simulink model "elec_sys_isolated"  (R2013b)
settings: Solver=ode45  StartTime=0.0  StopTime=10.0  RelTol=1e-3
values from neighbouring files (symbols this model uses):
  avload =     [Benchmark_data1.mat]
libraries: PowerFlowLib x28, simulink x5
settings Model: Creator=srikanthan  LastModifiedBy=srikanthan

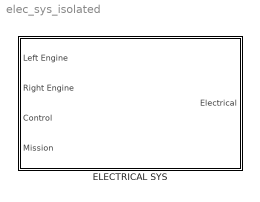
== system elec_sys_isolated ==
  "ELECTRICAL SYS " : Subsystem

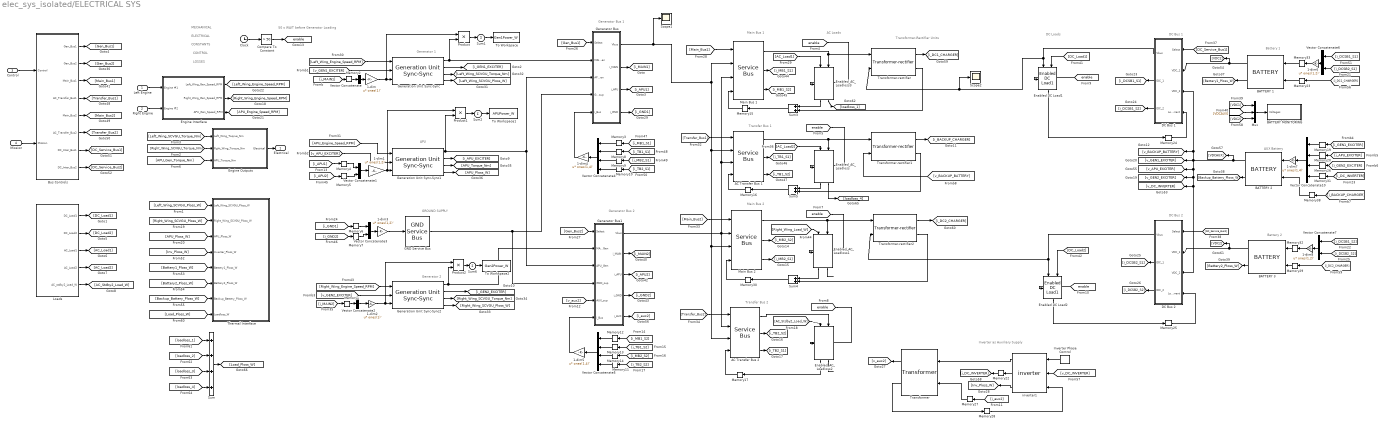
== system elec_sys_isolated/ELECTRICAL SYS  ==
  note: CONSTANTS
  note: CONTROL
  note: LOSSES
  note: MECHANICAL
  note: ELECTRICAL
  note: Generator Bus 1
  note: Generator 1
  note: APU
  note: GROUND SUPPLY
  note: Generator 2
  note: Main Bus 1
  note: Transfer Bus 1
  note: Main Bus 2
  note: Transfer Bus 2
  note: AC Loads
  note: Transformer-Rectifier Units
  note: DC Loads
  note: DC Bus 1
  note: DC Bus 2
  note: Battery 1
  note: AUX Battery
  note: Battery 2
  note: Inverter as Auxiliary Supply
  note: 50 s WAIT before Generator Loading
  note: Generator Bus 2
  Left Engine : Inport
  Right Engine : Inport  Port=2
  Control : Inport  Port=3
  Mission : Inport  Port=4
  " inverter1" : PowerFlowLib/Energy & Power Systems/Electrical/Inverters/ inverter  Trise=4e-6  Tfall=4e-6  fsw=2e3  Vcesat=1.2  Nofsw=6
  1-dim : Gain  Gain=ones(1)'  Multiplication=Matrix(u*K)
  1-dim{1,3,6,8} (4 alike) : Gain  Gain=ones(1,2)'  Multiplication=Matrix(u*K)
  1-dim2 : Gain  Gain=ones(1)'  Multiplication=Matrix(u*K)
  1-dim4 : Gain  Gain=ones(1,4)'  Multiplication=Matrix(u*K)
  1-dim5 : Gain  Gain=ones(1,4)'  Multiplication=Matrix(u*K)
  1-dim7 : Gain  Gain=ones(1,4)'  Multiplication=Matrix(u*K)
  AC Transfer Bus 1 : PowerFlowLib/Energy & Power Systems/Electrical/Systems/Service Bus
  AC Transfer Bus 2 : PowerFlowLib/Energy & Power Systems/Electrical/Systems/Service Bus
  BATTERY 1 : PowerFlowLib/Energy & Power Systems/Electrical/Battery/BATTERY  NO_CELLS=8  NO_MODULES=100  INITIAL_SOC=1
  BATTERY 2 : PowerFlowLib/Energy & Power Systems/Electrical/Battery/BATTERY  NO_CELLS=8  NO_MODULES=100  INITIAL_SOC=1
  BATTERY 3 : PowerFlowLib/Energy & Power Systems/Electrical/Battery/BATTERY  NO_CELLS=8  NO_MODULES=100  INITIAL_SOC=1
  BATTERY MONITORING : Subsystem  mask{mon_t=10}
      mask prompts: mon_t "Battery monitoring interval (s)"
  Bus Controls : Subsystem  mask{BUS1=Generator 1, BUS2=Generator 2, MBUS1=Generator Bus 1, ACTBUS1=Generator Bus 1, MBUS2=Generator Bus 2, ACTBUS2=Generator Bus 2, IDCBUS1=Battery 1, IDCBUS2=Battery 2}
      mask prompts: BUS1 "Source for Bus 1"; BUS2 "Source for Bus 2"; MBUS1 "Load on Main Bus 1 drawn from"; ACTBUS1 "Load on AC Transfer Bus 1 drawn from"; MBUS2 "Load on Main Bus 2 drawn from"; ACTBUS2 "Load on AC Transfer Bus 2 drawn from"; IDCBUS1 "Source for DC Service Bus 1"; IDCBUS2 "Source for DC Service Bus 2"
      mask help:
      | Specify the source from which different buses receive power. There are
      | 1. Two Generator buses (Bus 1-2)
      | 2. Two AC Main buses (Main Bus 1-2))
      | 3. Two AC Transfer buses and (AC Transfer Bus 1-2)
      | 4. Two DC Intermediate buses (DC Intermediate Bus 1-2)
      mask init:
      | switch BUS1
      |     case 1
      |         BUS1CONTROL = 1;
      |     case 2
      |         BUS1CONTROL = 2;
      |     case 3
      |         BUS1CONTROL = 3;
      |     case 4
      |         BUS1CONTROL = 4;
      | end
      | 
      | switch BUS2
      |     case 1
      |         BUS2CONTROL = 1;
      |     case 2
      |         BUS2CONTROL = 2;
      |     case 3
      |         BUS2CONTROL = 3;
      |     case 4
      |         BUS2CONTROL = 4;
      | end
      | 
      | switch MBUS1
      |     case 1
      |         MBUS1CONTROL = 1;
      |     case 2
      |         MBUS1CONTROL = 2;
      | end
      | 
      | switch ACTBUS1
      |     case 1
      |         ACTBUS1CONTROL = 1;
      |     case 2
      |         ACTBUS1CONTROL = 2;
      | end
      | 
      | switch MBUS2
      |     case 1
      |         MBUS2CONTROL = 1;
      |     case 2
      |         MBUS2CONTROL = 2;
      | end
      | 
      | switch ACTBUS2
      |     case 1
      |         ACTBUS2CONTROL = 1;
      |     case 2
      |         ACTBUS2CONTROL = 2;
      | end
      | 
      | switch IDCBUS1
      |     case 1
      |         IDCBUS1CONTROL = 1;
      |     case 2
      |         IDCBUS1CONTROL = 2;
      | end
      | 
      | switch IDCBUS2
      |     case 1
      |         IDCBUS2CONTROL = 1;
      |     case 2
      |         IDCBUS2CONTROL = 2;
      | end
      mask TypeOptions BUS1: Generator 1  | APU  | GND | AUX SUPPLY
      mask TypeOptions BUS2: Generator 2  | APU  | GND | AUX SUPPLY
      mask TypeOptions MBUS1: Generator Bus 1 | Generator Bus 2
      mask TypeOptions ACTBUS1: Generator Bus 1 | Generator Bus 2
      mask TypeOptions MBUS2: Generator Bus 1 | Generator Bus 2
      mask TypeOptions ACTBUS2: Generator Bus 1 | Generator Bus 2
      mask TypeOptions IDCBUS1: Battery 1 | Battery 2
      mask TypeOptions IDCBUS2: Battery 1 | Battery 2
  Clock : Clock
  Compare To Constant : simulink/Logic and Bit Operations/Compare To Constant  relop=>  const=50  OutDataTypeStr=uint8
  DC Bus 1 : Subsystem  mask(DC Service Bus){}
      mask help: Service Bus
  DC Bus 2 : Subsystem  mask(DC Service Bus){}
      mask help: Service Bus
  Enabled DC Load1 : PowerFlowLib/Energy & Power Systems/Electrical/Loads/Enabled  DC Load1
  Enabled DC Load2 : PowerFlowLib/Energy & Power Systems/Electrical/Loads/Enabled  DC Load1
  Enabled_AC_Loadloss : PowerFlowLib/Energy & Power Systems/Electrical/Loads/Enabled_AC_Loadloss  P=0  Q=0  E=0.98  ILRMS=0  R=10000  X=10000
  Enabled_AC_Loadloss1 : PowerFlowLib/Energy & Power Systems/Electrical/Loads/Enabled_AC_Loadloss  P=0  Q=0  E=0.98  ILRMS=0  R=10000  X=10000
  Enabled_AC_Loadloss2 : PowerFlowLib/Energy & Power Systems/Electrical/Loads/Enabled_AC_Loadloss  P=0  Q=0  E=0.98  ILRMS=0  R=10000  X=10000
  Enabled_AC_Loadloss3 : PowerFlowLib/Energy & Power Systems/Electrical/Loads/Enabled_AC_Loadloss  P=500  Q=500  E=0.98  ILRMS=0  R=10000  X=10000
  Engine Interface : Subsystem
  Engine Outputs : Subsystem
  GND Service Bus : PowerFlowLib/Energy & Power Systems/Electrical/Systems/GND Service Bus
  Generation Unit Sync-Sync : PowerFlowLib/Energy & Power Systems/Electrical/Systems/Generation Unit Sync-Sync  machine_mode=300kVA_Gen  init_gear='init_gear_box.mat'  fan_load='init_fan_characteristics.mat'  exciter_param='exciter.mat'
  Generation Unit Sync-Sync1 : PowerFlowLib/Energy & Power Systems/Electrical/Systems/Generation Unit Sync-Sync  machine_mode=300kVA_Gen  init_gear='init_gear_box.mat'  fan_load='init_fan_characteristics.mat'  exciter_param='exciter.mat'
  Generation Unit Sync-Sync2 : PowerFlowLib/Energy & Power Systems/Electrical/Systems/Generation Unit Sync-Sync  machine_mode=300kVA_Gen  init_gear='init_gear_box.mat'  fan_load='init_fan_characteristics.mat'  exciter_param='exciter.mat'
  Generator Bus : Subsystem
      mask help: Generator Bus Structure.
  Generator Bus1 : Subsystem
      mask help: Generator Bus Structure.
  Inverter Phase Control : PowerFlowLib/Energy & Power Systems/Electrical/Systems/Inverter Phase Control
  Loads : Subsystem  mask(Avionics load configuration){avopt=Read from .mat file, mean=100, var=20, sampt=20, initavload='initavload.mat'}
      mask prompts: avopt "Enter Avionics load :"; mean "Mean load in W:"; var "Variance:"; sampt "Sample interval:"; initavload "Enter pathname of the mat file to load :"
      mask init:
      | blk = gcb;
      | value = get_param(blk,'avopt');
      | 
      | if strcmp(value,'As average with variation')
      |      STATS = 1;
      | else
      |      STATS = 2;
      |      load('initavload.mat');
      | end
      | 
      | clear blk value
      mask TypeOptions avopt: As average with variation | Read from .mat file
      mask Callback avopt:
      | blk = gcb;
      | value = get_param(blk,'avopt');
      | 
      | if strcmp(value,'As average with variation')
      |      STATS = 1;
      |      cellarr(1:4)={'on'};
      |      cellarr(5)={'off'};
      | else
      |      STATS = 2;
      |       cellarr(1)={'on'};
      |      cellarr(2:4)={'off'};
      |      cellarr(5)={'on'};
      |      load('initavload.mat');
      |  end
      |  set_param(blk,'MaskVisibilities',cellarr);
      |  clear blk STATS value cellarr
  Main Bus 1 : PowerFlowLib/Energy & Power Systems/Electrical/Systems/Service Bus
  Main Bus 2 : PowerFlowLib/Energy & Power Systems/Electrical/Systems/Service Bus
  Memory{1..17,19..20,22..33,38} (32 alike) : Memory
  Mux : Mux  Inputs=3
  Product : Product
  Product1 : Product
  Product2 : Product
  Scope1 : Scope
      settings: YMin=295.01  YMax=295.013  SaveName=gevol
  Scope2 : Scope
      settings: YMin=295.01  YMax=295.013  SaveName=chgct
  Sum : Sum  Inputs=++++
  Sum1 : Sum  Inputs=+
  Sum2 : Sum  Inputs=+
  Sum3 : Sum
  Sum4 : Sum
  Sum5 : Sum
  Sum6 : Sum  Inputs=+
  Thermal Interface : Subsystem
  To Workspace : ToWorkspace  VariableName=Gen1Power_W  SampleTime=10  SaveFormat=Structure With Time
  To Workspace1 : ToWorkspace  VariableName=APUPower_W  SampleTime=10  SaveFormat=Structure With Time
  To Workspace2 : ToWorkspace  VariableName=Gen2Power_W  SampleTime=10  SaveFormat=Structure With Time
  Transformer : PowerFlowLib/Energy & Power Systems/Electrical/Machines/Transformer  Rp=0.005  Rs=0.1  N1=32  N2=120
  Transformer-rectifier : PowerFlowLib/Energy & Power Systems/Electrical/Systems/Transformer-rectifier  pu=1
  Transformer-rectifier1 : PowerFlowLib/Energy & Power Systems/Electrical/Systems/Transformer-rectifier  pu=1
  Transformer-rectifier2 : PowerFlowLib/Energy & Power Systems/Electrical/Systems/Transformer-rectifier  pu=1
  Vector Concatenate : Concatenate  NumInputs=1  Mode=Multidimensional array  ConcatenateDimension=2
  Vector Concatenate{1,3,6..7} (4 alike) : Concatenate  Mode=Multidimensional array  ConcatenateDimension=2
  Vector Concatenate10 : Concatenate  NumInputs=4  Mode=Multidimensional array  ConcatenateDimension=2
  Vector Concatenate2 : Concatenate  NumInputs=1  Mode=Multidimensional array  ConcatenateDimension=2
  Vector Concatenate4 : Concatenate  NumInputs=4  Mode=Multidimensional array  ConcatenateDimension=2
  Vector Concatenate5 : Concatenate  NumInputs=4  Mode=Multidimensional array  ConcatenateDimension=2
  Electrical : Outport
  tag scope: enable=global
  wires:
  [AC_Stdby2_Load_W] -> Enabled_AC_Loadloss2/1
  AC Transfer Bus 2/1 -> Enabled_AC_Loadloss2/2
  Enabled_AC_Loadloss2/1 -> Memory17/1
  Memory17/1 -> AC Transfer Bus 2/4
  BATTERY 2/1 -> [v_GEN1_EXCITER], [v_APU_EXCITER], [v_GEN2_EXCITER], [v_DC_INVERTER], DC Bus 2/3(VDC_2), [v_BACKUP_BATTERY], DC Bus 1/3(VDC_2), [VDCAUX]
  BATTERY 3/1 -> DC Bus 2/2(VDC_1), [VDC2]
  BATTERY 1/1 -> DC Bus 1/2(VDC_1), [VDC1]
  Generation Unit Sync-Sync/1 -> Product/2, Generator Bus/2(MAIN_Gen)
  GND Service Bus/1 -> Generator Bus/4(GND_sup), Generator Bus1/4(GND_sup)
  Generator Bus/3(i_APU) -> [i_APU1]
  Generator Bus/4(i_GND) -> [i_GND1]
  Vector Concatenate/1 -> 1-dim/1
  1-dim/1 -> Product/1, Generation Unit Sync-Sync/3
  Vector Concatenate1/1 -> 1-dim1/1
  Vector Concatenate3/1 -> 1-dim3/1
  1-dim3/1 -> GND Service Bus/1
  [Left_Wing_Engine_Speed_RPM] -> Generation Unit Sync-Sync/1
  [APU_Engine_Speed_RPM] -> Generation Unit Sync-Sync1/1
  [Gen_Bus1] -> Generator Bus/1(Select)
  Generator Bus/1(Vbus) -> Scope1/1, Main Bus 2/3, AC Transfer Bus 2/3, AC Transfer Bus 1/2, Main Bus 1/2
  [i_APU2] -> Memory5/1
  [i_GND2] -> Memory7/1
  [i_MAIN1] -> Memory2/1
  [i_APU1] -> Memory4/1
  [i_GND1] -> Memory6/1
  Memory2/1 -> Vector Concatenate/1
  Memory4/1 -> Vector Concatenate1/1
  Memory5/1 -> Vector Concatenate1/2
  Memory6/1 -> Vector Concatenate3/1
  Memory7/1 -> Vector Concatenate3/2
  Generator Bus/2(i_MAIN) -> [i_MAIN1]
  Generator Bus1/3(i_APU) -> [i_APU2]
  Generator Bus1/4(i_GND) -> [i_GND2]
  Generator Bus1/1(Vbus) -> Main Bus 1/3, AC Transfer Bus 1/3, Main Bus 2/2, AC Transfer Bus 2/2
  Generator Bus1/2(i_MAIN) -> [i_MAIN2]
  Vector Concatenate2/1 -> 1-dim2/1
  [i_MAIN2] -> Memory1/1
  Memory1/1 -> Vector Concatenate2/1
  Generation Unit Sync-Sync2/1 -> Product2/2, Generator Bus1/2(MAIN_Gen)
  [Gen_Bus2] -> Generator Bus1/1(Select)
  [Main_Bus1] -> Main Bus 1/1
  [Transfer_Bus1] -> AC Transfer Bus 1/1
  [Main_Bus2] -> Main Bus 2/1
  [Transfer_Bus2] -> AC Transfer Bus 2/1
  Main Bus 1/2 -> [i_MB1_S1]
  Main Bus 1/3 -> [i_MB1_S2]
  AC Transfer Bus 1/2 -> [i_TB1_S1]
  AC Transfer Bus 1/3 -> [i_TB1_S2]
  Main Bus 2/2 -> [i_MB2_S2]
  Main Bus 2/3 -> [i_MB2_S1]
  AC Transfer Bus 2/2 -> [i_TB2_S2]
  AC Transfer Bus 2/3 -> [i_TB2_S1]
  Main Bus 1/1 -> Transformer-rectifier/1, Enabled_AC_Loadloss3/2
  Memory15/1 -> Main Bus 1/4
  Memory16/1 -> AC Transfer Bus 1/4
  AC Transfer Bus 1/1 -> Transformer-rectifier1/1, Enabled_AC_Loadloss/2
  [AC_Load2] -> Enabled_AC_Loadloss/1
  Main Bus 2/1 -> Transformer-rectifier2/1, Enabled_AC_Loadloss1/2
  Memory30/1 -> Main Bus 2/4
  Generation Unit Sync-Sync/4 -> [Left_Wing_SCVGU_Ploss_W]
  Generation Unit Sync-Sync/3 -> [Left_Wing_SCVGU_Torque_Nm]
  Generation Unit Sync-Sync2/4 -> [Right_Wing_SCVGU_Ploss_W]
  Generation Unit Sync-Sync2/3 -> [Right_Wing_SCVGU_Torque_Nm]
  Generation Unit Sync-Sync1/3 -> [APU_Torque_Nm]
  Generation Unit Sync-Sync1/4 -> [APU_Ploss_W]
  [AC_Load1] -> Enabled_AC_Loadloss3/1
  [Right_Wing_Load_W] -> Enabled_AC_Loadloss1/1
  Engine Outputs/1(Electrical) -> Electrical/1
  [Left_Wing_SCVGU_Torque_Nm] -> Engine Outputs/1(Left_Wing_Toqrue_Nm)
  [Right_Wing_SCVGU_Torque_Nm] -> Engine Outputs/2(Rght_Wing_Torque_Nm)
  [APU_Gen_Torque_Nm] -> Engine Outputs/3(APU_Torque_Nm)
  Engine Interface/1(Left_Wing_Gen_Speed_RPM) -> [Left_Wing_Engine_Speed_RPM]
  Engine Interface/2(Right_Wing_Gen_Speed_RPM) -> [Right_Wing_Engine_Speed_RPM]
  Engine Interface/3(APU_Gen_Speed_RPM) -> [APU_Engine_Speed_RPM]
  DC Bus 1/1(Vbus) -> Scope2/1, Transformer-rectifier/2, Enabled DC Load1/1
  DC Bus 2/1(Vbus) -> Transformer-rectifier2/2, Enabled DC Load2/1
  Memory24/1 -> DC Bus 1/4(Load current)
  Memory25/1 -> DC Bus 2/4(Load current)
  [DC_Service_Bus1] -> DC Bus 1/1(Select)
  [DC_Service_Bus2] -> DC Bus 2/1(Select)
  [DC_Load1] -> Enabled DC Load1/2
  [DC_Load2] -> Enabled DC Load2/2
  DC Bus 1/2(IDC_1) -> [i_DCSB1_S1]
  DC Bus 1/3(IDC_2) -> [i_DCSB1_S2]
  DC Bus 2/2(IDC_1) -> [i_DCSB2_S1]
  DC Bus 2/3(IDC_2) -> [i_DCSB2_S2]
  BATTERY 1/2 -> [Battery1_Ploss_W]
  BATTERY 2/2 -> [Backup_Battery_Ploss_W]
  BATTERY 3/2 -> [Battery2_Ploss_W]
  Left Engine/1 -> Engine Interface/1(Engine #1)
  Right Engine/1 -> Engine Interface/2(Engine #2)
  [v_GEN1_EXCITER] -> Generation Unit Sync-Sync/2
  Generation Unit Sync-Sync/2 -> [i_GEN1_EXCITER]
  [v_APU_EXCITER] -> Generation Unit Sync-Sync1/2
  Generation Unit Sync-Sync1/2 -> [i_APU_EXCITER]
  [Right_Wing_Engine_Speed_RPM] -> Generation Unit Sync-Sync2/1
  [v_GEN2_EXCITER] -> Generation Unit Sync-Sync2/2
  Generation Unit Sync-Sync2/2 -> [i_GEN2_EXCITER]
  Enabled DC Load2/1 -> Memory25/1
  Memory27/1 -> Transformer/2
  Transformer-rectifier/2 -> Sum3/2
  Sum3/1 -> Memory15/1
  Enabled_AC_Loadloss3/1 -> Sum3/1
  Sum4/1 -> Memory30/1
  Enabled_AC_Loadloss1/1 -> Sum4/1
  Sum5/1 -> Memory16/1
  Enabled_AC_Loadloss/1 -> Sum5/1
  Transformer-rectifier1/1 -> [i_BACKUP_CHARGER]
  Clock/1 -> Compare To Constant/1
  Compare To Constant/1 -> [enable]
  [enable] -> Enabled_AC_Loadloss2/Enable
  [enable] -> Enabled DC Load1/Enable
  [enable] -> Enabled DC Load2/Enable
  Transformer/2 -> Memory28/1
  Transformer/1 -> [v_aux2]
  [v_aux2] -> Generator Bus1/5(AUX_sup)
  Generator Bus1/5(i_AUX) -> [i_aux2]
  " inverter1"/3 -> [Inv_Ploss_W]
  Memory28/1 -> " inverter1"/3
  " inverter1"/1 -> Transformer/1
  Inverter Phase Control/1 -> " inverter1"/1
  [v_DC_INVERTER] -> " inverter1"/2
  " inverter1"/2 -> Memory22/1
  Memory22/1 -> [i_DC_INVERTER]
  [i_aux2] -> Memory27/1
  [v_BACKUP_BATTERY] -> Transformer-rectifier1/2
  Transformer-rectifier1/2 -> Sum5/2
  Transformer-rectifier2/2 -> Sum4/2
  [enable] -> Enabled_AC_Loadloss/Enable
  [enable] -> Enabled_AC_Loadloss1/Enable
  [enable] -> Enabled_AC_Loadloss3/Enable
  Bus Controls/7(DC_Inter_Bus1) -> [DC_Service_Bus1]
  Bus Controls/8(DC_Inter_Bus2) -> [DC_Service_Bus2]
  Bus Controls/1(Gen_Bus1) -> [Gen_Bus1]
  Bus Controls/2(Gen_Bus2) -> [Gen_Bus2]
  Bus Controls/3(Main_Bus1) -> [Main_Bus1]
  Bus Controls/4(AC_Transfer_Bus1) -> [Transfer_Bus1]
  Bus Controls/5(Main_Bus2) -> [Main_Bus2]
  Bus Controls/6(AC_Transfer_Bus2) -> [Transfer_Bus2]
  Mission/1 -> Bus Controls/2(Mission)
  Control/1 -> Bus Controls/1(Control)
  Memory3/1 -> Vector Concatenate4/1
  Memory8/1 -> Vector Concatenate4/2
  Memory9/1 -> Vector Concatenate4/3
  Memory10/1 -> Vector Concatenate4/4
  [i_MB1_S1] -> Memory3/1
  [i_TB1_S1] -> Memory8/1
  [i_MB2_S1] -> Memory9/1
  [i_TB2_S1] -> Memory10/1
  Vector Concatenate4/1 -> 1-dim4/1
  1-dim4/1 -> Generator Bus/5(i_Bus)
  Memory12/1 -> Vector Concatenate5/1
  Memory13/1 -> Vector Concatenate5/2
  Memory14/1 -> Vector Concatenate5/3
  Memory11/1 -> Vector Concatenate5/4
  [i_MB1_S2] -> Memory12/1
  [i_TB1_S2] -> Memory13/1
  [i_MB2_S2] -> Memory14/1
  [i_TB2_S2] -> Memory11/1
  Vector Concatenate5/1 -> 1-dim5/1
  1-dim5/1 -> Generator Bus1/6(i_Bus)
  Loads/1(DC_Load1) -> [DC_Load1]
  Loads/2(DC_Load2) -> [DC_Load2]
  Loads/3(AC_Load1) -> [AC_Load1]
  Loads/4(AC_Load2) -> [AC_Load2]
  Loads/5(AC_stdby2_Load_W) -> [AC_Stdby2_Load_W]
  Memory33/1 -> BATTERY 1/1
  Memory23/1 -> BATTERY 1/2
  1-dim6/1 -> Memory33/1
  [i_DCSB1_S1] -> Vector Concatenate6/1
  [i_DCSB2_S1] -> Vector Concatenate6/2
  Vector Concatenate6/1 -> 1-dim6/1
  [i_DC1_CHARGER] -> Memory23/1
  Vector Concatenate10/1 -> 1-dim7/1
  1-dim7/1 -> BATTERY 2/1
  [i_GEN1_EXCITER] -> Memory19/1
  [i_APU_EXCITER] -> Memory20/1
  [i_GEN2_EXCITER] -> Memory26/1
  Memory38/1 -> BATTERY 2/2
  [i_BACKUP_CHARGER] -> Memory38/1
  Memory26/1 -> Vector Concatenate10/3
  Memory20/1 -> Vector Concatenate10/2
  Memory19/1 -> Vector Concatenate10/1
  Memory31/1 -> Vector Concatenate10/4
  [i_DC_INVERTER] -> Memory31/1
  Memory32/1 -> BATTERY 3/1
  1-dim8/1 -> Memory32/1
  [i_DCSB1_S2] -> Vector Concatenate7/1
  [i_DCSB2_S2] -> Vector Concatenate7/2
  Vector Concatenate7/1 -> 1-dim8/1
  Memory29/1 -> BATTERY 3/2
  [i_DC2_CHARGER] -> Memory29/1
  Transformer-rectifier/1 -> [i_DC1_CHARGER]
  Transformer-rectifier2/1 -> [i_DC2_CHARGER]
  Enabled DC Load1/1 -> Memory24/1
  Mux/1 -> BATTERY MONITORING/1(Voltages)
  [VDC1] -> Mux/1
  [VDCAUX] -> Mux/2
  [VDC2] -> Mux/3
  [Left_Wing_SCVGU_Ploss_W] -> Thermal Interface/1(Left_Wing_SCVGU_Ploss_W)
  [Right_Wing_SCVGU_Ploss_W] -> Thermal Interface/2(Right_Wing_SCVGU_Ploss_W)
  [APU_Ploss_W] -> Thermal Interface/3(APU_Ploss_W)
  [Inv_Ploss_W] -> Thermal Interface/4(Inverter_Ploss_W)
  [Battery1_Ploss_W] -> Thermal Interface/5(Battery1_Ploss_W)
  [Battery2_Ploss_W] -> Thermal Interface/6(Battery2_Ploss_W)
  [Backup_Battery_Ploss_W] -> Thermal Interface/7(Backup_Battery_Ploss_W)
  [Load_Ploss_W] -> Thermal Interface/8(Loadloss_W)
  [loadloss_1] -> Sum/1
  [loadloss_2] -> Sum/2
  [loadloss_3] -> Sum/3
  [loadloss_4] -> Sum/4
  Sum/1 -> [Load_Ploss_W]
  Enabled_AC_Loadloss3/2 -> [loadloss_1]
  Enabled_AC_Loadloss1/2 -> ?
  Enabled_AC_Loadloss2/2 -> ?
  Enabled_AC_Loadloss/2 -> [loadloss_4]
  Product/1 -> Sum1/1
  Sum1/1 -> To Workspace/1
  Generation Unit Sync-Sync1/1 -> Product1/2, Generator Bus/3(APU_Gen), Generator Bus1/3(APU_Gen)
  1-dim1/1 -> Product1/1, Generation Unit Sync-Sync1/3
  Product1/1 -> Sum2/1
  Sum2/1 -> To Workspace1/1
  1-dim2/1 -> Product2/1, Generation Unit Sync-Sync2/3
  Product2/1 -> Sum6/1
  Sum6/1 -> To Workspace2/1

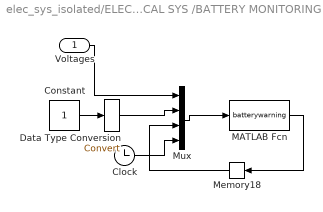
== system elec_sys_isolated/ELECTRICAL SYS /BATTERY MONITORING ==
  Voltages : Inport
  Clock : Clock
  Constant : Constant
  Data Type Conversion : DataTypeConversion
  MATLAB Fcn : MATLABFcn  MATLABFcn=batterywarning  SampleTime=mon_t
  Memory18 : Memory  X0=[0 0 0]
  Mux : Mux
  wires:
  Mux/1 -> MATLAB Fcn/1
  MATLAB Fcn/1 -> Memory18/1
  Memory18/1 -> Mux/3
  Constant/1 -> Data Type Conversion/1
  Voltages/1 -> Mux/1
  Data Type Conversion/1 -> Mux/2
  Clock/1 -> Mux/4

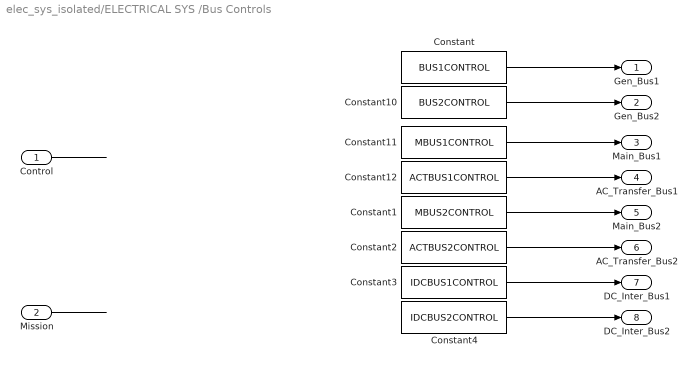
== system elec_sys_isolated/ELECTRICAL SYS /Bus Controls ==
  Control : Inport
  Mission : Inport  Port=2
  Constant : Constant  Value=BUS1CONTROL
  Constant1 : Constant  Value=MBUS2CONTROL
  Constant10 : Constant  Value=BUS2CONTROL
  Constant11 : Constant  Value=MBUS1CONTROL
  Constant12 : Constant  Value=ACTBUS1CONTROL
  Constant2 : Constant  Value=ACTBUS2CONTROL
  Constant3 : Constant  Value=IDCBUS1CONTROL
  Constant4 : Constant  Value=IDCBUS2CONTROL
  Gen_Bus1 : Outport
  Gen_Bus2 : Outport  Port=2
  Main_Bus1 : Outport  Port=3
  AC_Transfer_Bus1 : Outport  Port=4
  Main_Bus2 : Outport  Port=5
  AC_Transfer_Bus2 : Outport  Port=6
  DC_Inter_Bus1 : Outport  Port=7
  DC_Inter_Bus2 : Outport  Port=8
  wires:
  Constant/1 -> Gen_Bus1/1
  Constant10/1 -> Gen_Bus2/1
  Constant11/1 -> Main_Bus1/1
  Constant12/1 -> AC_Transfer_Bus1/1
  Constant1/1 -> Main_Bus2/1
  Constant2/1 -> AC_Transfer_Bus2/1
  Constant3/1 -> DC_Inter_Bus1/1
  Constant4/1 -> DC_Inter_Bus2/1
  Mission/1 -> ?
  Control/1 -> ?

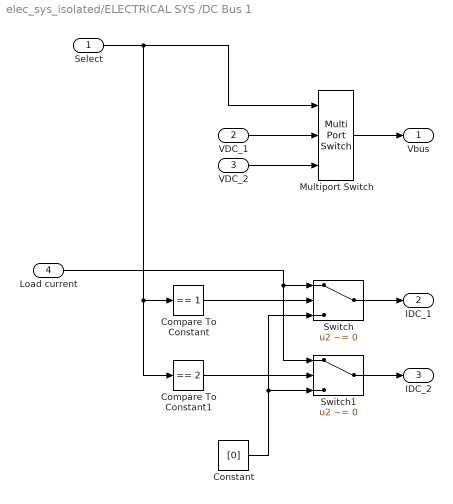
== system elec_sys_isolated/ELECTRICAL SYS /DC Bus 1 ==
  Select : Inport
  VDC_1 : Inport  Port=2
  VDC_2 : Inport  Port=3
  Load current : Inport  Port=4
  Compare To Constant : simulink/Logic and Bit Operations/Compare To Constant  relop===  const=1  OutDataTypeStr=uint8
  Compare To Constant1 : simulink/Logic and Bit Operations/Compare To Constant  relop===  const=2  OutDataTypeStr=uint8
  Constant : Constant  Value=[0]
  Multiport Switch : MultiPortSwitch  Inputs=2
  Switch : Switch  Criteria=u2 ~= 0
  Switch1 : Switch  Criteria=u2 ~= 0
  Vbus : Outport
  IDC_1 : Outport  Port=2
  IDC_2 : Outport  Port=3
  wires:
  Load current/1 -> Switch1/1, Switch/1
  Multiport Switch/1 -> Vbus/1
  VDC_1/1 -> Multiport Switch/2
  VDC_2/1 -> Multiport Switch/3
  Select/1 -> Multiport Switch/1, Compare To Constant/1, Compare To Constant1/1
  Compare To Constant/1 -> Switch/2
  Compare To Constant1/1 -> Switch1/2
  Constant/1 -> Switch/3, Switch1/3
  Switch/1 -> IDC_1/1
  Switch1/1 -> IDC_2/1

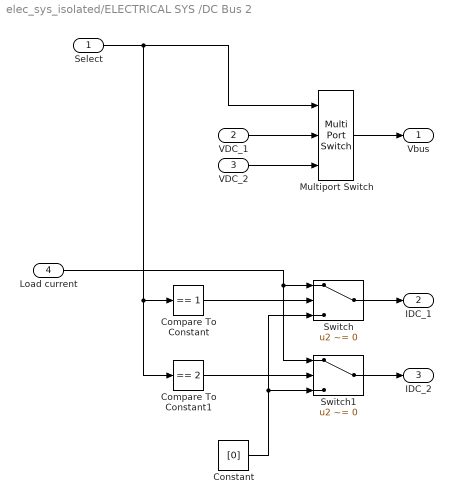
== system elec_sys_isolated/ELECTRICAL SYS /DC Bus 2 ==
  Select : Inport
  VDC_1 : Inport  Port=2
  VDC_2 : Inport  Port=3
  Load current : Inport  Port=4
  Compare To Constant : simulink/Logic and Bit Operations/Compare To Constant  relop===  const=1  OutDataTypeStr=uint8
  Compare To Constant1 : simulink/Logic and Bit Operations/Compare To Constant  relop===  const=2  OutDataTypeStr=uint8
  Constant : Constant  Value=[0]
  Multiport Switch : MultiPortSwitch  Inputs=2
  Switch : Switch  Criteria=u2 ~= 0
  Switch1 : Switch  Criteria=u2 ~= 0
  Vbus : Outport
  IDC_1 : Outport  Port=2
  IDC_2 : Outport  Port=3
  wires:
  Switch1/1 -> IDC_2/1
  Switch/1 -> IDC_1/1
  Constant/1 -> Switch1/3, Switch/3
  Compare To Constant1/1 -> Switch1/2
  Compare To Constant/1 -> Switch/2
  Select/1 -> Compare To Constant1/1, Compare To Constant/1, Multiport Switch/1
  VDC_2/1 -> Multiport Switch/3
  VDC_1/1 -> Multiport Switch/2
  Multiport Switch/1 -> Vbus/1
  Load current/1 -> Switch/1, Switch1/1

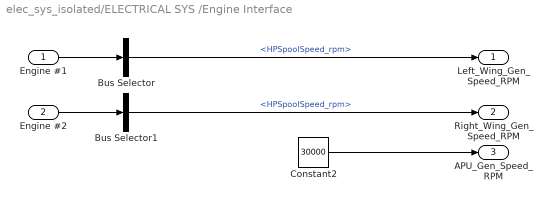
== system elec_sys_isolated/ELECTRICAL SYS /Engine Interface ==
  Engine #1 : Inport
  Engine #2 : Inport  Port=2
  Bus Selector : BusSelector  OutputSignals=Spools.HPSpoolSpeed_rpm
  Bus Selector1 : BusSelector  OutputSignals=Spools.HPSpoolSpeed_rpm
  Constant2 : Constant  Value=30000
  Left_Wing_Gen_Speed_RPM : Outport
  Right_Wing_Gen_Speed_RPM : Outport  Port=2
  APU_Gen_Speed_RPM : Outport  Port=3
  wires:
  Constant2/1 -> APU_Gen_Speed_RPM/1
  Bus Selector1/1 -> Right_Wing_Gen_Speed_RPM/1  "<HPSpoolSpeed_rpm>"
  Bus Selector/1 -> Left_Wing_Gen_Speed_RPM/1  "<HPSpoolSpeed_rpm>"
  Engine #1/1 -> Bus Selector/1
  Engine #2/1 -> Bus Selector1/1

== system elec_sys_isolated/ELECTRICAL SYS /Engine Outputs ==
  Left_Wing_Toqrue_Nm : Inport
  Rght_Wing_Torque_Nm : Inport  Port=2
  APU_Torque_Nm : Inport  Port=3
  Bus Creator : BusCreator  Inputs=3
  Electrical : Outport
  wires:
  Rght_Wing_Torque_Nm/1 -> Bus Creator/2  "Right Wing Torq (Nm)"
  APU_Torque_Nm/1 -> Bus Creator/3  "APU Torq (Nm)"
  Left_Wing_Toqrue_Nm/1 -> Bus Creator/1  "Left Wing Torq (Nm)"
  Bus Creator/1 -> Electrical/1

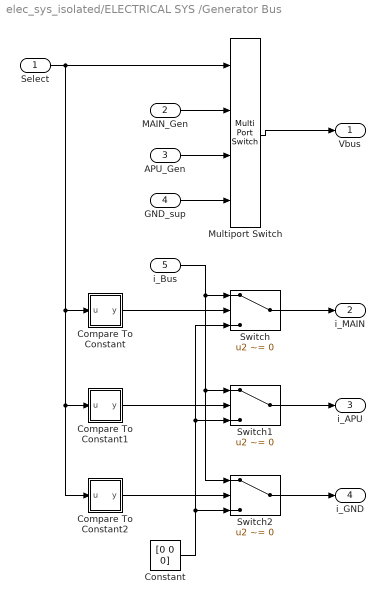
== system elec_sys_isolated/ELECTRICAL SYS /Generator Bus ==
  Select : Inport
  MAIN_Gen : Inport  Port=2
  APU_Gen : Inport  Port=3
  GND_sup : Inport  Port=4
  i_Bus : Inport  Port=5
  Compare To Constant : Subsystem  mask(Compare To Constant){relop===, const=1, LogicOutDataTypeMode=uint8, ZeroCross=on}
      mask prompts: relop "Operator:"; const "Constant value:"; LogicOutDataTypeMode "Output data type mode:"; ZeroCross "Enable zero-crossing detection"
      mask help: Determine how a signal compares to a constant.
      mask init:
      | blkName = gcb;
      | 
      | if strcmp(get_param(gcbh,'LogicOutDataTypeMode'),'boolean')
      | 	setValue = 'Boolean';
      | else
      | 	setValue = 'Specify via dialog';
      | end
      | 
      | set_param([blkName,'/Compare'],'relop',relop, ...
      | 	'LogicOutDataTypeMode', setValue, 'ZeroCross', ZeroCross);
      | 
      | str = [relop,' C']; %default
      | 
      | const_str = get_param(blkName, 'const');
      | 
      | if isempty(strfind(const_str, ' ')) && isempty(strfind(const_str, ','))
      |     % scalar or single expression
      |     if isempty(str2num(const_str))
      |         %expression
      |         str = [relop, ' ', const_str];
      |     elseif length(const) == 1
      |         str = [relop,' ',num2str(double(const))];
      |     end
      | end
      mask TypeOptions relop: == | ~= | < | <= | >= | >
      mask TypeOptions LogicOutDataTypeMode: uint8 | boolean
      mask Callback ZeroCross: sl('zeroCrossEnable', gcbh);
      mask Display: disp(str)
  Compare To Constant1 : Subsystem  mask(Compare To Constant){relop===, const=2, LogicOutDataTypeMode=uint8, ZeroCross=on}
      mask prompts: relop "Operator:"; const "Constant value:"; LogicOutDataTypeMode "Output data type mode:"; ZeroCross "Enable zero-crossing detection"
      mask help: Determine how a signal compares to a constant.
      mask init: same as elec_sys_isolated/ELECTRICAL SYS /Generator Bus/Compare To Constant
      mask TypeOptions relop: == | ~= | < | <= | >= | >
      mask TypeOptions LogicOutDataTypeMode: uint8 | boolean
      mask Callback ZeroCross: sl('zeroCrossEnable', gcbh);
      mask Display: disp(str)
  Compare To Constant2 : Subsystem  mask(Compare To Constant){relop===, const=3, LogicOutDataTypeMode=uint8, ZeroCross=on}
      mask prompts: relop "Operator:"; const "Constant value:"; LogicOutDataTypeMode "Output data type mode:"; ZeroCross "Enable zero-crossing detection"
      mask help: Determine how a signal compares to a constant.
      mask init: same as elec_sys_isolated/ELECTRICAL SYS /Generator Bus/Compare To Constant
      mask TypeOptions relop: == | ~= | < | <= | >= | >
      mask TypeOptions LogicOutDataTypeMode: uint8 | boolean
      mask Callback ZeroCross: sl('zeroCrossEnable', gcbh);
      mask Display: disp(str)
  Constant : Constant  Value=[0 0 0]
  Multiport Switch : MultiPortSwitch
  Switch : Switch  Criteria=u2 ~= 0  Threshold=0.5
  Switch1 : Switch  Criteria=u2 ~= 0  Threshold=0.5
  Switch2 : Switch  Criteria=u2 ~= 0  Threshold=0.5
  Vbus : Outport
  i_MAIN : Outport  Port=2
  i_APU : Outport  Port=3
  i_GND : Outport  Port=4
  wires:
  MAIN_Gen/1 -> Multiport Switch/2
  APU_Gen/1 -> Multiport Switch/3
  GND_sup/1 -> Multiport Switch/4
  Multiport Switch/1 -> Vbus/1
  Select/1 -> Multiport Switch/1, Compare To Constant/1(u), Compare To Constant2/1(u), Compare To Constant1/1(u)
  Switch/1 -> i_MAIN/1
  Switch1/1 -> i_APU/1
  Switch2/1 -> i_GND/1
  i_Bus/1 -> Switch/1, Switch2/1, Switch1/1
  Compare To Constant/1(y) -> Switch/2
  Compare To Constant1/1(y) -> Switch1/2
  Compare To Constant2/1(y) -> Switch2/2
  Constant/1 -> Switch2/3, Switch1/3, Switch/3

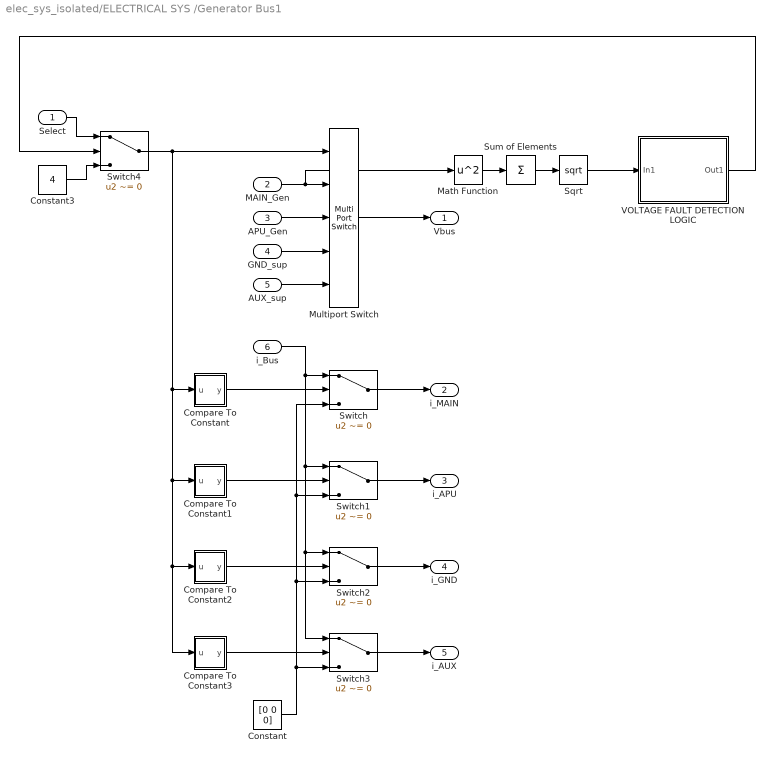
== system elec_sys_isolated/ELECTRICAL SYS /Generator Bus1 ==
  Select : Inport
  MAIN_Gen : Inport  Port=2
  APU_Gen : Inport  Port=3
  GND_sup : Inport  Port=4
  AUX_sup : Inport  Port=5
  i_Bus : Inport  Port=6
  Compare To Constant : Subsystem  mask(Compare To Constant){relop===, const=1, LogicOutDataTypeMode=uint8, ZeroCross=on}
      mask prompts: relop "Operator:"; const "Constant value:"; LogicOutDataTypeMode "Output data type mode:"; ZeroCross "Enable zero-crossing detection"
      mask help: Determine how a signal compares to a constant.
      mask init: same as elec_sys_isolated/ELECTRICAL SYS /Generator Bus/Compare To Constant
      mask TypeOptions relop: == | ~= | < | <= | >= | >
      mask TypeOptions LogicOutDataTypeMode: uint8 | boolean
      mask Callback ZeroCross: sl('zeroCrossEnable', gcbh);
      mask Display: disp(str)
  Compare To Constant1 : Subsystem  mask(Compare To Constant){relop===, const=2, LogicOutDataTypeMode=uint8, ZeroCross=on}
      mask prompts: relop "Operator:"; const "Constant value:"; LogicOutDataTypeMode "Output data type mode:"; ZeroCross "Enable zero-crossing detection"
      mask help: Determine how a signal compares to a constant.
      mask init: same as elec_sys_isolated/ELECTRICAL SYS /Generator Bus/Compare To Constant
      mask TypeOptions relop: == | ~= | < | <= | >= | >
      mask TypeOptions LogicOutDataTypeMode: uint8 | boolean
      mask Callback ZeroCross: sl('zeroCrossEnable', gcbh);
      mask Display: disp(str)
  Compare To Constant2 : Subsystem  mask(Compare To Constant){relop===, const=3, LogicOutDataTypeMode=uint8, ZeroCross=on}
      mask prompts: relop "Operator:"; const "Constant value:"; LogicOutDataTypeMode "Output data type mode:"; ZeroCross "Enable zero-crossing detection"
      mask help: Determine how a signal compares to a constant.
      mask init: same as elec_sys_isolated/ELECTRICAL SYS /Generator Bus/Compare To Constant
      mask TypeOptions relop: == | ~= | < | <= | >= | >
      mask TypeOptions LogicOutDataTypeMode: uint8 | boolean
      mask Callback ZeroCross: sl('zeroCrossEnable', gcbh);
      mask Display: disp(str)
  Compare To Constant3 : Subsystem  mask(Compare To Constant){relop===, const=4, LogicOutDataTypeMode=uint8, ZeroCross=on}
      mask prompts: relop "Operator:"; const "Constant value:"; LogicOutDataTypeMode "Output data type mode:"; ZeroCross "Enable zero-crossing detection"
      mask help: Determine how a signal compares to a constant.
      mask init: same as elec_sys_isolated/ELECTRICAL SYS /Generator Bus/Compare To Constant
      mask TypeOptions relop: == | ~= | < | <= | >= | >
      mask TypeOptions LogicOutDataTypeMode: uint8 | boolean
      mask Callback ZeroCross: sl('zeroCrossEnable', gcbh);
      mask Display: disp(str)
  Constant : Constant  Value=[0 0 0]
  Constant3 : Constant  Value=4
  Math Function : Math  Operator=square  SaturateOnIntegerOverflow=on
  Multiport Switch : MultiPortSwitch  Inputs=4
  Sqrt : Sqrt  SaturateOnIntegerOverflow=on
  Sum of Elements : Sum  Inputs=+
  Switch{,1..4} (5 alike) : Switch  Criteria=u2 ~= 0  Threshold=0.5
  VOLTAGE FAULT DETECTION LOGIC : Subsystem
  Vbus : Outport
  i_MAIN : Outport  Port=2
  i_APU : Outport  Port=3
  i_GND : Outport  Port=4
  i_AUX : Outport  Port=5
  wires:
  Constant/1 -> Switch/3, Switch1/3, Switch2/3, Switch3/3
  Compare To Constant3/1(y) -> Switch3/2
  Compare To Constant2/1(y) -> Switch2/2
  Compare To Constant1/1(y) -> Switch1/2
  Compare To Constant/1(y) -> Switch/2
  i_Bus/1 -> Switch3/1, Switch2/1, Switch1/1, Switch/1
  Switch3/1 -> i_AUX/1
  Switch2/1 -> i_GND/1
  Switch1/1 -> i_APU/1
  Switch/1 -> i_MAIN/1
  Switch4/1 -> Compare To Constant3/1(u), Compare To Constant2/1(u), Compare To Constant1/1(u), Compare To Constant/1(u), Multiport Switch/1
  Multiport Switch/1 -> Vbus/1
  AUX_sup/1 -> Multiport Switch/5
  GND_sup/1 -> Multiport Switch/4
  APU_Gen/1 -> Multiport Switch/3
  MAIN_Gen/1 -> Multiport Switch/2, Math Function/1
  Select/1 -> Switch4/1
  Constant3/1 -> Switch4/3
  VOLTAGE FAULT DETECTION LOGIC/1(Out1) -> Switch4/2
  Math Function/1 -> Sum of Elements/1
  Sum of Elements/1 -> Sqrt/1
  Sqrt/1 -> VOLTAGE FAULT DETECTION LOGIC/1(In1)

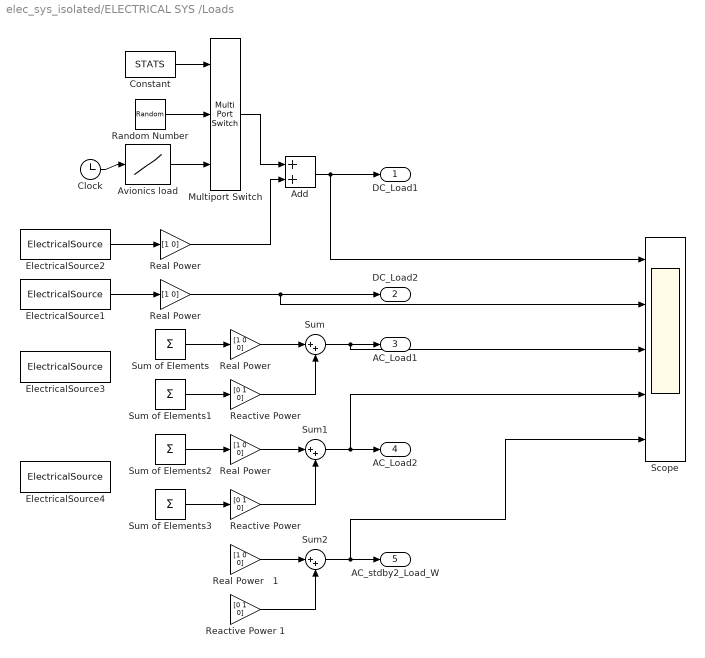
== system elec_sys_isolated/ELECTRICAL SYS /Loads ==
  Add : Sum
  Avionics load : Lookup  InputValues=avload.time  Table=avload.load
  Clock : Clock
  Constant : Constant  Value=STATS
  ElectricalSource1 : PowerFlowLib/Support Functions//Tools/ElectricalSource  Tag=Flow  Description=TwoPhase  load_loc=Cabin  ACDC_load=DC
  ElectricalSource2 : PowerFlowLib/Support Functions//Tools/ElectricalSource  Tag=Flow  Description=TwoPhase  load_loc=Cockpit  ACDC_load=DC
  ElectricalSource3 : PowerFlowLib/Support Functions//Tools/ElectricalSource  Tag=Flow  Description=TwoPhase  load_loc=RightWing  ACDC_load=AC
  ElectricalSource4 : PowerFlowLib/Support Functions//Tools/ElectricalSource  Tag=Flow  Description=TwoPhase  load_loc=LeftWing  ACDC_load=AC
  Multiport Switch : MultiPortSwitch  Inputs=2  DiagnosticForDefault=Warning
  Random Number : RandomNumber  Mean=mean  Variance=var  SampleTime=sampt
  Reactive Power : Gain  Gain=[0 1 0]
  "Reactive Power " : Gain  Gain=[0 1 0]
  Reactive Power 1 : Gain  Gain=[0 1 0]
  Real Power : Gain  Gain=[1 0]
  "Real Power " : Gain  Gain=[1 0]
  "Real Power  " : Gain  Gain=[1 0 0]
  "Real Power   " : Gain  Gain=[1 0 0]
  Real Power   1 : Gain  Gain=[1 0 0]
  Scope : Scope  NumInputPorts=5
      settings: YMin=-1~-1~0~0~-1  YMax=1~1~125000~125000~1  SaveName=ScopeData31  SampleInput=on  SampleTime=1
  Sum : Sum  Inputs=|++
  Sum of Elements{,1..3} (4 alike) : Sum  Inputs=+
  Sum1 : Sum  Inputs=|++
  Sum2 : Sum  Inputs=|++
  DC_Load1 : Outport
  DC_Load2 : Outport  Port=2
  AC_Load1 : Outport  Port=3
  AC_Load2 : Outport  Port=4
  AC_stdby2_Load_W : Outport  Port=5
  wires:
  ? -> Sum of Elements3/1
  ? -> Sum of Elements2/1
  ? -> Sum of Elements1/1
  ElectricalSource1/1 -> "Real Power "/1
  Real Power   1/1 -> Sum2/1
  Reactive Power 1/1 -> Sum2/2
  Sum2/1 -> AC_stdby2_Load_W/1, Scope/5
  ElectricalSource2/1 -> Real Power/1
  "Real Power  "/1 -> Sum/1
  Reactive Power/1 -> Sum/2
  "Real Power   "/1 -> Sum1/1
  "Reactive Power "/1 -> Sum1/2
  Sum/1 -> AC_Load1/1, Scope/3
  Sum1/1 -> AC_Load2/1, Scope/4
  "Real Power "/1 -> DC_Load2/1, Scope/2
  ? -> Sum of Elements/1
  Sum of Elements/1 -> "Real Power  "/1
  Sum of Elements1/1 -> Reactive Power/1
  Sum of Elements2/1 -> "Real Power   "/1
  Sum of Elements3/1 -> "Reactive Power "/1
  Random Number/1 -> Multiport Switch/2
  Constant/1 -> Multiport Switch/1
  Avionics load/1 -> Multiport Switch/3
  Clock/1 -> Avionics load/1
  Multiport Switch/1 -> Add/1
  Real Power/1 -> Add/2
  Add/1 -> DC_Load1/1, Scope/1

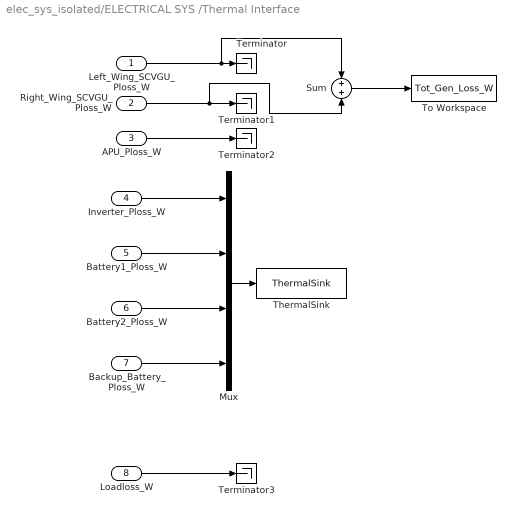
== system elec_sys_isolated/ELECTRICAL SYS /Thermal Interface ==
  Left_Wing_SCVGU_Ploss_W : Inport
  Right_Wing_SCVGU_Ploss_W : Inport  Port=2
  APU_Ploss_W : Inport  Port=3
  Inverter_Ploss_W : Inport  Port=4
  Battery1_Ploss_W : Inport  Port=5
  Battery2_Ploss_W : Inport  Port=6
  Backup_Battery_Ploss_W : Inport  Port=7
  Loadloss_W : Inport  Port=8
  Mux : Mux
  Sum : Sum
  Terminator{,1..3} (4 alike) : Terminator
  ThermalSink : PowerFlowLib/Support Functions//Tools/ThermalSink  Tag=Flow  Description=TwoPhase  load_loc=Cabin  units=Watts  unq_id=8332
  To Workspace : ToWorkspace  VariableName=Tot_Gen_Loss_W  SampleTime=10  SaveFormat=Structure With Time
  wires:
  Right_Wing_SCVGU_Ploss_W/1 -> Sum/2, Terminator1/1
  APU_Ploss_W/1 -> Terminator2/1
  Mux/1 -> ThermalSink/1
  Inverter_Ploss_W/1 -> Mux/1
  Battery1_Ploss_W/1 -> Mux/2
  Battery2_Ploss_W/1 -> Mux/3
  Backup_Battery_Ploss_W/1 -> Mux/4
  Loadloss_W/1 -> Terminator3/1
  Left_Wing_SCVGU_Ploss_W/1 -> Sum/1, Terminator/1
  Sum/1 -> To Workspace/1

== system elec_sys_isolated/ELECTRICAL SYS /Generator Bus/Compare To Constant ==
  u : Inport
  Compare : RelationalOperator  Operator===  OutDataTypeStr=fixdt(0, 8)  InputSameDT=on
  Constant : Constant  DisableCoverage=on  Value=const  OutDataTypeStr=Inherit: Inherit via back propagation
  y : Outport
  wires:
  u/1 -> Compare/1
  Constant/1 -> Compare/2
  Compare/1 -> y/1

== system elec_sys_isolated/ELECTRICAL SYS /Generator Bus/Compare To Constant1 ==
  u : Inport
  Compare : RelationalOperator  Operator===  OutDataTypeStr=fixdt(0, 8)  InputSameDT=on
  Constant : Constant  DisableCoverage=on  Value=const  OutDataTypeStr=Inherit: Inherit via back propagation
  y : Outport
  wires:
  u/1 -> Compare/1
  Constant/1 -> Compare/2
  Compare/1 -> y/1

== system elec_sys_isolated/ELECTRICAL SYS /Generator Bus/Compare To Constant2 ==
  u : Inport
  Compare : RelationalOperator  Operator===  OutDataTypeStr=fixdt(0, 8)  InputSameDT=on
  Constant : Constant  DisableCoverage=on  Value=const  OutDataTypeStr=Inherit: Inherit via back propagation
  y : Outport
  wires:
  u/1 -> Compare/1
  Constant/1 -> Compare/2
  Compare/1 -> y/1

== system elec_sys_isolated/ELECTRICAL SYS /Generator Bus1/Compare To Constant ==
  u : Inport
  Compare : RelationalOperator  Operator===  OutDataTypeStr=fixdt(0, 8)  InputSameDT=on
  Constant : Constant  DisableCoverage=on  Value=const  OutDataTypeStr=Inherit: Inherit via back propagation
  y : Outport
  wires:
  Compare/1 -> y/1
  Constant/1 -> Compare/2
  u/1 -> Compare/1

== system elec_sys_isolated/ELECTRICAL SYS /Generator Bus1/Compare To Constant1 ==
  u : Inport
  Compare : RelationalOperator  Operator===  OutDataTypeStr=fixdt(0, 8)  InputSameDT=on
  Constant : Constant  DisableCoverage=on  Value=const  OutDataTypeStr=Inherit: Inherit via back propagation
  y : Outport
  wires:
  Compare/1 -> y/1
  Constant/1 -> Compare/2
  u/1 -> Compare/1

== system elec_sys_isolated/ELECTRICAL SYS /Generator Bus1/Compare To Constant2 ==
  u : Inport
  Compare : RelationalOperator  Operator===  OutDataTypeStr=fixdt(0, 8)  InputSameDT=on
  Constant : Constant  DisableCoverage=on  Value=const  OutDataTypeStr=Inherit: Inherit via back propagation
  y : Outport
  wires:
  Compare/1 -> y/1
  Constant/1 -> Compare/2
  u/1 -> Compare/1

== system elec_sys_isolated/ELECTRICAL SYS /Generator Bus1/Compare To Constant3 ==
  u : Inport
  Compare : RelationalOperator  Operator===  OutDataTypeStr=fixdt(0, 8)  InputSameDT=on
  Constant : Constant  DisableCoverage=on  Value=const  OutDataTypeStr=Inherit: Inherit via back propagation
  y : Outport
  wires:
  Compare/1 -> y/1
  Constant/1 -> Compare/2
  u/1 -> Compare/1

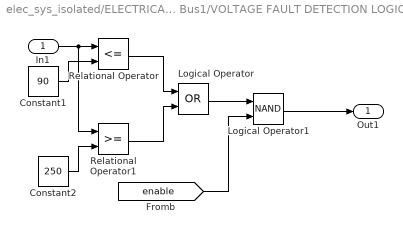
== system elec_sys_isolated/ELECTRICAL SYS /Generator Bus1/VOLTAGE FAULT DETECTION LOGIC ==
  In1 : Inport
  Constant1 : Constant  Value=90
  Constant2 : Constant  Value=250
  Logical Operator : Logic  Operator=OR  AllPortsSameDT=off  OutDataTypeStr=boolean
  Logical Operator1 : Logic  Operator=NAND  AllPortsSameDT=off  OutDataTypeStr=boolean
  Relational Operator : RelationalOperator  Operator=<=  OutDataTypeStr=boolean  ZeroCross=off
  Relational Operator1 : RelationalOperator  OutDataTypeStr=boolean  ZeroCross=off
  Out1 : Outport
  wires:
  Constant1/1 -> Relational Operator/2
  Constant2/1 -> Relational Operator1/2
  Relational Operator/1 -> Logical Operator/1
  Relational Operator1/1 -> Logical Operator/2
  Logical Operator/1 -> Logical Operator1/1
  [enable] -> Logical Operator1/2
  In1/1 -> Relational Operator/1, Relational Operator1/1
  Logical Operator1/1 -> Out1/1
